simulink library "WheelSlipControl_Lib"  (R2019b)
settings: Solver=VariableStepAuto  StartTime=0.0  StopTime=10.0  RelTol=1e-3  EnableMultiTasking=on
libraries: simulink x4, LatchesLib x2, TimersLib x1
settings Model: Creator=cdyer  LastModifiedBy=mondt
settings DataIOCC: LimitDataPoints=on
settings OptimizationCC: LifeSpan=inf
settings DebuggingCC: AllowSymbolicDim=off  SFUnexpectedBacktrackingDiag=warning  SFNoUnconditionalDefaultTransitionDiag=warning  SFExecutionAtInitializationDiag=none  ArithmeticOperatorsInVariantConditions=warning
settings ModelReferenceCC: PropagateSignalLabelsOutOfModel=off
settings SFSimCC: SimUseLocalCustomCode=off  CustomCodeUndefinedFunction=UseInterfaceOnly
settings RTWCC: RTWUseLocalCustomCode=off
settings CodeAppCC: StateflowObjectComments=on
settings GRTTargetCC: TargetLangStandard=C89/C90 (ANSI)
settings ConfigComp: CovMetricSettings=dw  CovHtmlReporting=on  CovSaveCumulativeToWorkspaceVar=on  CovSaveSingleToWorkspaceVar=on  CovExternalEMLEnable=off

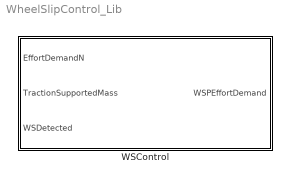
== system WheelSlipControl_Lib ==
  WSControl : Subsystem  mask(Wheel Slip/Slide Control){JerkLim=0.6}
      mask prompts: JerkLim "Jerk Limit (acceleration or deceleration) [m/s3]"
      mask help:
      | When slip/slide detected, tractive/braking effort is dropped by equivalent of 2x jerk limit
      | When slip/slide no longer detected, tractive/braking effort is increased at jerk limit back to demanded level
      | If slip/slide is detected again during the recovery of tractive/braking effort, the traction/braking effort will still increase despite the slip/slide, but only at half the jerk limit, until adhesion is restored.
      mask Display:
      | plot([0.1, 0.2, 0.25, 0.4, 0.5, 0.55, 0.625, 0.625, 0.8], [0.7, 0.7, 0.3, 0.7, 0.7, 0.3, 0.55, 0.5, 0.7]);
      | plot([0.1, 0.1], [0.0, 0.9])
      | plot([0.0, 0.9], [0.1, 0.1])
      | plot([0.0, 0.0], [0.0, 1.0])
      | plot([0.0, 1.0], [0.0, 0.0])
      | text(0.05, 0.95, 'N')
      | text(0.95, 0.1, 't')

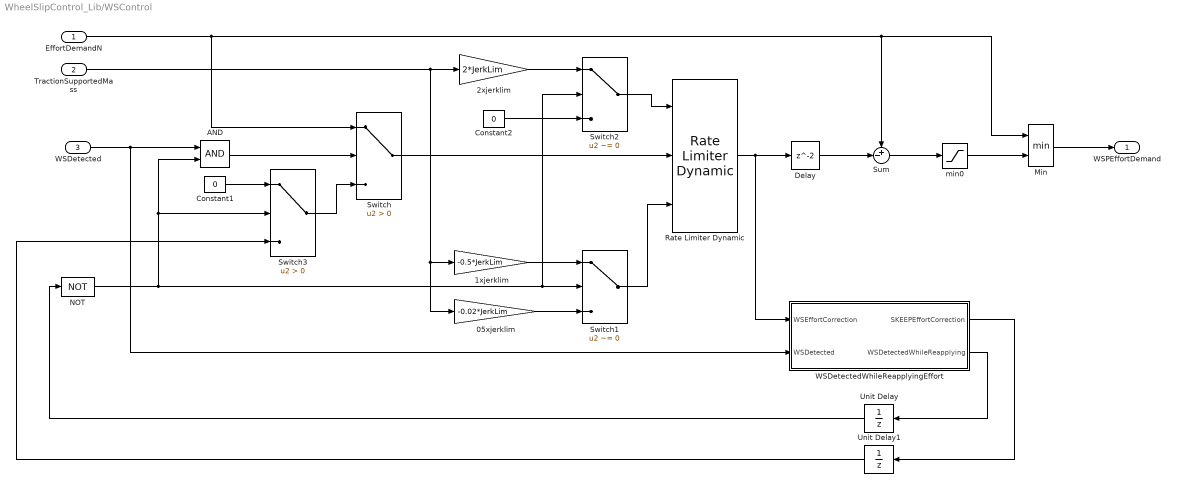
== system WheelSlipControl_Lib/WSControl ==
  EffortDemandN : Inport
  TractionSupportedMass : Inport  Port=2
  WSDetected : Inport  Port=3
  05xjerklim : Gain  Gain=-0.02*JerkLim
  1xjerklim : Gain  Gain=-0.5*JerkLim
  2xjerklim : Gain  Gain=2*JerkLim
  AND : Logic  AllPortsSameDT=off  OutDataTypeStr=boolean
  Constant1 : Constant  Value=0
  Constant2 : Constant  Value=0
  Delay : Delay
  Min : MinMax  Inputs=2
  NOT : Logic  Operator=NOT  AllPortsSameDT=off  OutDataTypeStr=boolean
  Rate Limiter Dynamic : simulink/Discontinuities/Rate Limiter Dynamic
      settings: SourceProductName=Simulink
  Sum : Sum  Inputs=+-|
  Switch : Switch  Criteria=u2 > Threshold
  Switch1 : Switch  Criteria=u2 ~= 0
  Switch2 : Switch  Criteria=u2 ~= 0
  Switch3 : Switch  Criteria=u2 > Threshold
  Unit Delay : UnitDelay  SampleTime=-1  HasFrameUpgradeWarning=on
  Unit Delay1 : UnitDelay  SampleTime=-1  HasFrameUpgradeWarning=on
  WSDetectedWhileReapplyingEffort : Subsystem
  min0 : Saturate  UpperLimit=inf  LowerLimit=0
  WSPEffortDemand : Outport
  wires:
  EffortDemandN/1 -> Min/1, Sum/1, Switch/1
  AND/1 -> Switch/2
  05xjerklim/1 -> Switch1/3
  Constant2/1 -> Switch2/3
  Min/1 -> WSPEffortDemand/1
  min0/1 -> Min/2
  Rate Limiter Dynamic/1 -> Delay/1, WSDetectedWhileReapplyingEffort/1(WSEffortCorrection)
  2xjerklim/1 -> Switch2/1
  1xjerklim/1 -> Switch1/1
  Sum/1 -> min0/1
  Switch/1 -> Rate Limiter Dynamic/2
  TractionSupportedMass/1 -> 2xjerklim/1, 1xjerklim/1, 05xjerklim/1
  WSDetected/1 -> AND/1, WSDetectedWhileReapplyingEffort/2(WSDetected)
  WSDetectedWhileReapplyingEffort/2(WSDetectedWhileReapplying) -> Unit Delay/1
  Unit Delay/1 -> NOT/1
  NOT/1 -> Switch3/2, AND/2, Switch2/2, Switch1/2
  Switch1/1 -> Rate Limiter Dynamic/3
  Switch2/1 -> Rate Limiter Dynamic/1
  Delay/1 -> Sum/2
  Constant1/1 -> Switch3/1
  Switch3/1 -> Switch/3
  WSDetectedWhileReapplyingEffort/1(SKEEPEffortCorrection) -> Unit Delay1/1
  Unit Delay1/1 -> Switch3/3

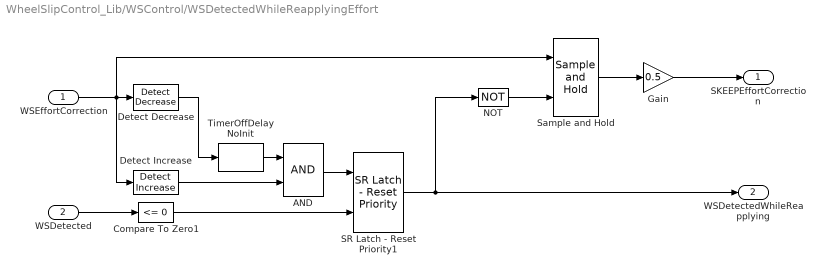
== system WheelSlipControl_Lib/WSControl/WSDetectedWhileReapplyingEffort ==
  WSEffortCorrection : Inport
  WSDetected : Inport  Port=2
  AND : Logic  AllPortsSameDT=off  OutDataTypeStr=boolean
  Compare To Zero1 : simulink/Logic and Bit Operations/Compare To Zero  relop=<=  OutDataTypeStr=boolean
  Detect Decrease : simulink/Logic and Bit Operations/Detect Decrease  vinit=0.0  OutDataTypeStr=boolean
  Detect Increase : simulink/Logic and Bit Operations/Detect Increase  vinit=0.0  OutDataTypeStr=boolean
  Gain : Gain  Gain=0.5
  NOT : Logic  Operator=NOT  AllPortsSameDT=off  OutDataTypeStr=boolean
  SR Latch - Reset Priority1 : LatchesLib/SR Latch - Reset Priority  initial_condition=0
      settings: SourceProductName=Latches
  Sample and Hold : LatchesLib/Sample and Hold  InitialCondition=0  SampleTime=-1
      settings: SourceProductName=Latches
  TimerOffDelay NoInit : TimersLib/TimerOffDelay NoInit  UpperSaturationLimit=0.1  SampleTime=-1
      settings: SourceProductName=Sydac Utilities
  SKEEPEffortCorrection : Outport
  WSDetectedWhileReapplying : Outport  Port=2
  wires:
  WSDetected/1 -> Compare To Zero1/1
  SR Latch - Reset Priority1/1 -> NOT/1, WSDetectedWhileReapplying/1
  WSEffortCorrection/1 -> Sample and Hold/1, Detect Increase/1, Detect Decrease/1
  Detect Decrease/1 -> TimerOffDelay NoInit/1
  Compare To Zero1/1 -> SR Latch - Reset Priority1/2
  AND/1 -> SR Latch - Reset Priority1/1
  Detect Increase/1 -> AND/2
  TimerOffDelay NoInit/1 -> AND/1
  NOT/1 -> Sample and Hold/2
  Sample and Hold/1 -> Gain/1
  Gain/1 -> SKEEPEffortCorrection/1
